simulink model "truck_parking_control"  (R2019a)
settings: Solver=FixedStepAuto  StartTime=0.0  StopTime=10  RelTol=1e-3
settings Model: Creator=ZISHUO  LastModifiedBy=ZISHUO

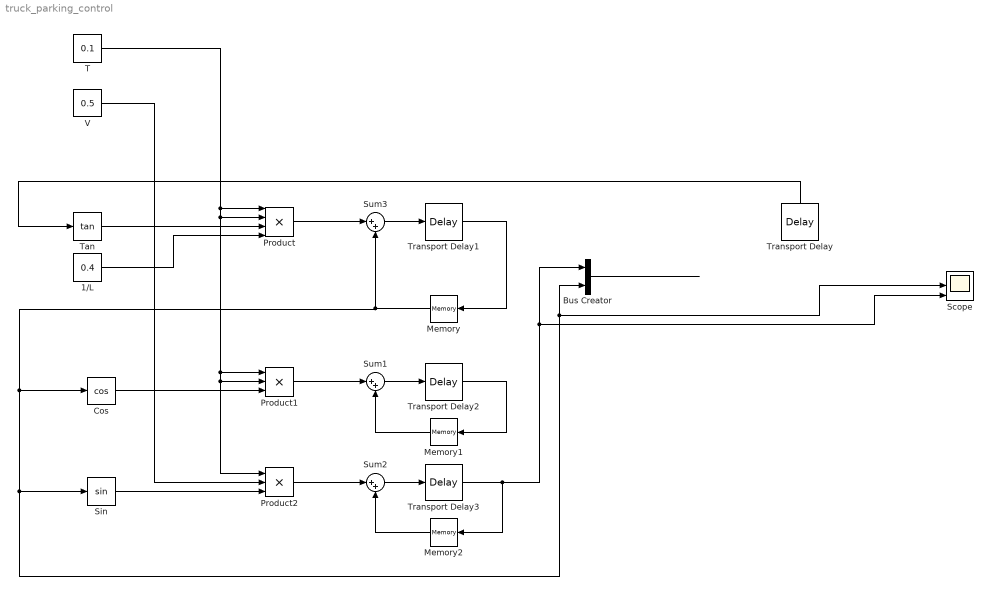
== system truck_parking_control ==
  " V" : Constant  Value=0.5
  1/L : Constant  Value=0.4
  Bus Creator : BusCreator  Inputs=2
  Cos : Trigonometry  Operator=cos
  Memory : Memory
  Memory1 : Memory  InitialCondition=20
  Memory2 : Memory  InitialCondition=40
  Product : Product  Inputs=4
  Product1 : Product  Inputs=3
  Product2 : Product  Inputs=3
  Scope : Scope  NumInputPorts=3
  Sin : Trigonometry
  Sum1 : Sum  Inputs=|++
  Sum2 : Sum  Inputs=|++
  Sum3 : Sum  Inputs=|++
  T : Constant  Value=0.1
  Tan : Trigonometry  Operator=tan
  Transport Delay{,1..3} (4 alike) : TransportDelay
  wires:
  ? -> Scope/1, Transport Delay/1
  1/L/1 -> Product/4
  Tan/1 -> Product/3
  T/1 -> Product/1, Product/2, Product1/1, Product1/2, Product2/1
  " V"/1 -> Product2/2
  Sin/1 -> Product2/3
  Cos/1 -> Product1/3
  Product2/1 -> Sum2/1
  Product1/1 -> Sum1/1
  Sum1/1 -> Transport Delay2/1
  Transport Delay2/1 -> Memory1/1
  Sum2/1 -> Transport Delay3/1
  Transport Delay3/1 -> Scope/3, Bus Creator/1, Memory2/1
  Product/1 -> Sum3/1
  Sum3/1 -> Transport Delay1/1
  Transport Delay1/1 -> Memory/1
  Transport Delay/1 -> Tan/1
  Memory/1 -> Cos/1, Sin/1, Scope/2, Bus Creator/2, Sum3/2
  Memory1/1 -> Sum1/2
  Memory2/1 -> Sum2/2
  Bus Creator/1 -> ?
